simulink model "S1_DHRLs"  (R2025b)
settings: Solver=ode1be  StartTime=0.0  StopTime=0.5  RelTol=1e-3
values from neighbouring files (symbols this model uses):
  a = 10    [S1_DHRL.m]
  b = 60    [S1_DHRL.m]
  b1 = 1.2611    [S1_DHRL.m]    (also in S1_sat.m)
  b2 = 0.8909    [S1_DHRL.m]    (also in S1_sat.m)
  c1 = 15.0914    [S1_DHRL.m]    (also in S1_sat.m)
  c2 = 13.4548    [S1_DHRL.m]    (also in S1_sat.m)
  gamma = 0.5508    [S1_DHRL.m]    (also in S1_sat.m)
  h = 0.001    [S1_DHRL.m]    (also in S1_sat.m)
  k = 21.9999    [S1_DHRL.m]    (also in S1_sat.m)
  k3 = 22.5    [S1_DHRL.m]
  k4 = 7.5    [S1_DHRL.m]
  Mb = 1.999*10^-4    (= 0.0001999)    [S1_DHRL.m]    (also in S1_sat.m)
  q1 = 3    [S1_DHRL.m]
  q2 = 3    [S1_DHRL.m]
  q3 = 3    [S1_DHRL.m]
undefined symbols (not defined in the file or in its folder): magnitude
libraries: fod x6
settings Model: Creator=IT7  LastModifiedBy=Wassim DJ

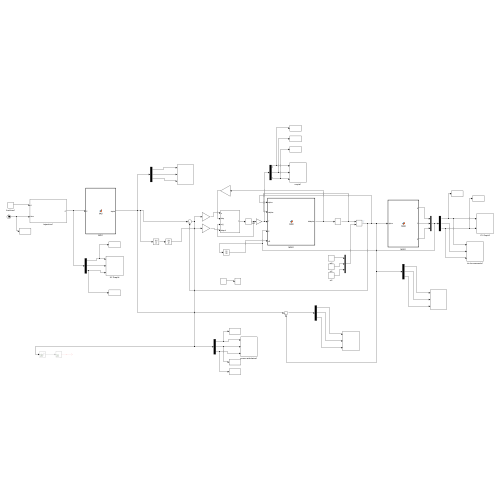
[thumbnail: Simulink's stored preview of the top-level diagram]
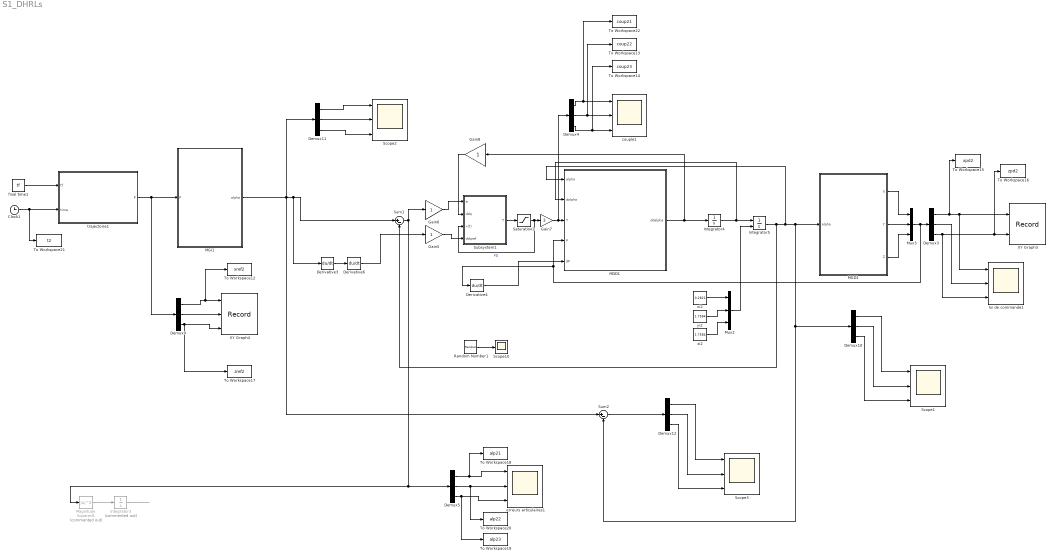
== system S1_DHRLs ==
  Clock1 : Clock
  Demux{3..5,9..12} (7 alike) : Demux  Outputs=3
  Derivative3 : Derivative
  Derivative4 : Derivative
  Derivative6 : Derivative
  Gain5 : Gain
  Gain6 : Gain
  Gain7 : Gain  Gain=3
  Gain8 : Gain
  Integrator3 : Integrator  Commented=on  InitialCondition=[0 0 0]
  Integrator4 : Integrator
  Integrator5 : Integrator  InitialConditionSource=external
  MDD1 : MATLAB Function  TreatAsAtomicUnit=on
  MGD1 : MATLAB Function  TreatAsAtomicUnit=on
  MGI1 : MATLAB Function  TreatAsAtomicUnit=on
  Magnitude Squared1 : Math  Commented=on  Operator=magnitude^2
  Mux2 : Mux  Inputs=3
  Mux3 : Mux  Inputs=3
  Random Number1 : RandomNumber  Variance=0.001  Seed=4  SampleTime=0.001
  Saturation2 : Saturate  UpperLimit=15/12  LowerLimit=-15/12
  Scope1 : Scope  NumInputPorts=3
      settings: ActiveDisplayYMinimum=-0.04767  ActiveDisplayYMaximum=2.22139
  Scope10 : Scope
      settings: ActiveDisplayYMinimum=-0.11225  ActiveDisplayYMaximum=0.1102  DataLoggingVariableName=ScopeData2
  Scope2 : Scope  NumInputPorts=3
      settings: ActiveDisplayYMinimum=-0.0501  ActiveDisplayYMaximum=2.21858  DataLoggingVariableName=ScopeData3
  Scope3 : Scope  NumInputPorts=3
      settings: ActiveDisplayYMinimum=-0.00704  ActiveDisplayYMaximum=0.00073  DataLoggingVariableName=ScopeData4
  Subsystem1 : Subsystem
  Sum1 : Sum  Inputs=|+-
  Sum2 : Sum  Inputs=|+-
  To Workspace12 : ToWorkspace  VariableName=xref2  SampleTime=-1
      settings: Save2DSignal=2-D array (concatenate along first dimension)
  To Workspace13 : ToWorkspace  VariableName=coup22  SampleTime=-1
      settings: Save2DSignal=2-D array (concatenate along first dimension)
  To Workspace14 : ToWorkspace  VariableName=coup23  SampleTime=-1
      settings: Save2DSignal=2-D array (concatenate along first dimension)
  To Workspace15 : ToWorkspace  VariableName=xpd2  SampleTime=-1
      settings: Save2DSignal=2-D array (concatenate along first dimension)
  To Workspace16 : ToWorkspace  VariableName=zpd2  SampleTime=-1
      settings: Save2DSignal=2-D array (concatenate along first dimension)
  To Workspace17 : ToWorkspace  VariableName=zref2  SampleTime=-1
      settings: Save2DSignal=2-D array (concatenate along first dimension)
  To Workspace18 : ToWorkspace  VariableName=alp21  SampleTime=-1
      settings: Save2DSignal=2-D array (concatenate along first dimension)
  To Workspace19 : ToWorkspace  VariableName=alp23  SampleTime=-1
      settings: Save2DSignal=2-D array (concatenate along first dimension)
  To Workspace20 : ToWorkspace  VariableName=alp22  SampleTime=-1
      settings: Save2DSignal=2-D array (concatenate along first dimension)
  To Workspace21 : ToWorkspace  VariableName=t2  SampleTime=-1
      settings: Save2DSignal=2-D array (concatenate along first dimension)
  To Workspace22 : ToWorkspace  VariableName=coup21  SampleTime=-1
      settings: Save2DSignal=2-D array (concatenate along first dimension)
  XY Graph3 : Record  NumPorts=2.0  FileSettingsInternal="{\"entries\":[{\"content\":{\"excelSettings\":{\"content\":{},\"type\":\"Streamout.ExcelSettings\"},\"parquetSettings\":{\"content\":{},\"type\":\"Streamout.ParquetSettings\"}},\"type\":\"Streamout.FileSettingStorage\",\"uuid\":\"\"}],\"packageUris\":[\"http:\\/\\/schema.mathworks.com\\/mf0\\/streamout_blocks\\/R2020a\"],\"version\":\"1.0\"}"  FrameSettings=[0, 0]  Layout=[1 1]  SignalsInternal="{\"entries\":[{\"content\":{\"signals\":[{\"content\":{\"blockPath\":[],\"dimensions\":[1],\"domain\":\"\",\"lineColor\":\"#edb120\",\"lineWidth\":2,\"port\":1,\"signalID\":1,\"signalName\":\"Demux3:1\"},\"type\":\"RecordBlkView.Signal\",\"uuid\":\"\"},{\"content\":{\"blockPath\":[],\"dimensions\":[1],\"domain\":\"\",\"lineColor\":\"#7e2f8e\",\"lineWidth\":2,\"port\":2,\"signalID\":2,\"signalName\":\"Demux3:3\"},\"type\":\"RecordBlkView.Signal\",\"uuid\":\"\"}]},\"type\":\"RecordBlkView.InputSignals\",\"uuid\":\"\"}],\"packageUris\":[\"http:\\/\\/schema.mathworks.com\\/mf0\\/streamout_blocks\\/R2020a\"],\"version\":\"1.0\"}"  VisualizationBindings="{\"xyplotplugin\":{\"info\":[{\"series\":[],\"subplotID\":1}]}}"  CompatibilityTag=XY  st=-1
  XY Graph4 : Record  NumPorts=3.0  FileSettingsInternal="{\"entries\":[{\"content\":{\"excelSettings\":{\"content\":{},\"type\":\"Streamout.ExcelSettings\"},\"parquetSettings\":{\"content\":{},\"type\":\"Streamout.ParquetSettings\"}},\"type\":\"Streamout.FileSettingStorage\",\"uuid\":\"\"}],\"packageUris\":[\"http:\\/\\/schema.mathworks.com\\/mf0\\/streamout_blocks\\/R2020a\"],\"version\":\"1.0\"}"  FrameSettings=[0, 0, 0]  Layout=[1 1]  SignalsInternal="{\"entries\":[{\"content\":{\"signals\":[{\"content\":{\"blockPath\":[],\"dimensions\":[1,1],\"domain\":\"\",\"lineColor\":\"#77ac30\",\"lineWidth\":2,\"port\":1,\"signalID\":1,\"signalName\":\"Demux9:1\"},\"type\":\"RecordBlkView.Signal\",\"uuid\":\"\"},{\"content\":{\"blockPath\":[],\"dimensions\":[1,1],\"domain\":\"\",\"lineColor\":\"#4dbeee\",\"lineWidth\":2,\"port\":2,\"signalID\":2,\"signalName\":\"Demux9:2\"},\"type\":\"RecordBlkView.Signal\",\"uuid\":\"\"},{\"content\":{\"blockPath\":[],\"dimensions\":[1,1],\"domain\":\"\",\"lineColor\":\"#a2142f\",\"lineWidth\":2,\"port\":3,\"signalID\":3,\"signalName\":\"Demux9:3\"},\"type\":\"RecordBlkView.Signal\",\"uuid\":\"\"}]},\"type\":\"RecordBlkView.InputSignals\",\"uuid\":\"\"}],\"packageUris\":[\"http:\\/\\/schema.mathworks.com\\/mf0\\/streamout_blocks\\/R2020a\"],\"version\":\"1.0\"}"  VisualizationBindings="{\"xyplotplugin\":{\"info\":[{\"series\":[],\"subplotID\":1}]}}"  CompatibilityTag=XY  st=-1
  couple1 : Scope  NumInputPorts=3
      settings: ActiveDisplayYMinimum=-10.50451  ActiveDisplayYMaximum=10.07629  DataLoggingVariableName=ScopeData5
  erreurs articulaires1 : Scope  NumInputPorts=3
      settings: ActiveDisplayYMinimum=-0.00893  ActiveDisplayYMaximum=0.00194  DataLoggingVariableName=ScopeData6
  final time1 : Constant  Value=tf
  loi de commande1 : Scope  NumInputPorts=3
      settings: ActiveDisplayYMinimum=-0.50497  ActiveDisplayYMaximum=0.51496
  trajectoire1 : Subsystem
  xi2 : Constant  Value=0.2821
  yi2 : Constant  Value=1.7584
  zi2 : Constant  Value=1.7584
  wires:
  Integrator3/1 -> ?
  Demux12/2 -> Scope3/2
  xi2/1 -> Mux2/1
  Demux11/3 -> Scope2/3
  yi2/1 -> Mux2/2
  Subsystem1/1(T) -> Saturation2/1
  Demux12/3 -> Scope3/3
  Demux10/3 -> Scope1/3
  Demux3/1 -> XY Graph3/1, loi de commande1/1, To Workspace15/1
  Demux5/2 -> To Workspace20/1, erreurs articulaires1/2
  Demux4/1 -> To Workspace22/1, couple1/1
  Gain5/1 -> Subsystem1/4(ddqref)
  Gain8/1 -> Subsystem1/2(ddq)
  Derivative6/1 -> Gain5/1
  Mux2/1 -> Integrator5/2
  Derivative4/1 -> MDD1/5(dP)
  Random Number1/1 -> Scope10/1
  zi2/1 -> Mux2/3
  Sum2/1 -> Demux12/1
  Demux11/2 -> Scope2/2
  Gain7/1 -> Demux4/1, MDD1/3(T)
  Demux9/3 -> XY Graph4/3, To Workspace17/1
  trajectoire1/1(P) -> Demux9/1, MGI1/1(P)
  Demux9/1 -> To Workspace12/1, XY Graph4/1
  Demux11/1 -> Scope2/1
  Demux5/1 -> To Workspace18/1, erreurs articulaires1/1
  Derivative3/1 -> Derivative6/1
  final time1/1 -> trajectoire1/1(tf)
  Demux10/2 -> Scope1/2
  Integrator5/1 -> Sum1/2, MDD1/1(alpha), MGD1/1(alpha), Demux10/1, Sum2/2
  MDD1/1(ddalpha) -> Gain8/1, Integrator4/1
  MGD1/2(Y) -> Mux3/2
  MGD1/1(X) -> Mux3/1
  MGI1/1(alpha) -> Derivative3/1, Sum1/1, Sum2/1, Demux11/1
  Saturation2/1 -> Subsystem1/3(x(t)), Gain7/1  "PD"
  Demux9/2 -> XY Graph4/2
  Integrator4/1 -> MDD1/2(dalpha), Integrator5/1
  Demux4/3 -> To Workspace14/1, couple1/3
  Demux4/2 -> To Workspace13/1, couple1/2
  Demux10/1 -> Scope1/1
  Sum1/1 -> Magnitude Squared1/1, Demux5/1, Gain6/1
  Demux3/2 -> loi de commande1/2
  Magnitude Squared1/1 -> Integrator3/1
  Clock1/1 -> To Workspace21/1, trajectoire1/2("time ")
  Gain6/1 -> Subsystem1/1(e)
  MGD1/3(Z) -> Mux3/3
  Demux3/3 -> loi de commande1/3, XY Graph3/2, To Workspace16/1
  Mux3/1 -> MDD1/4(P), Derivative4/1, Demux3/1
  Demux5/3 -> To Workspace19/1, erreurs articulaires1/3
  Demux12/1 -> Scope3/1

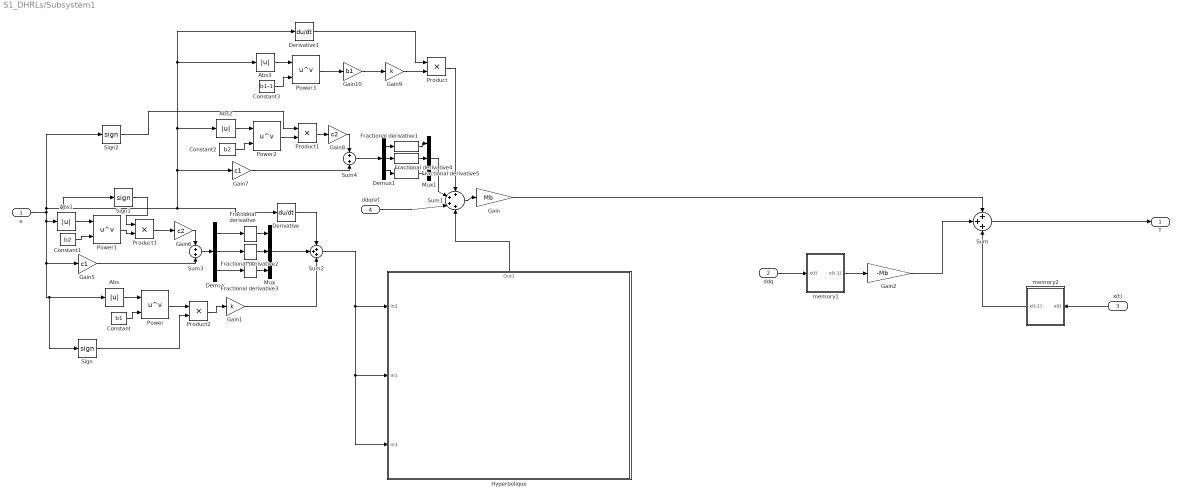
== system S1_DHRLs/Subsystem1 ==
  e : Inport
  ddq : Inport  Port=2
  x(t) : Inport  Port=3
  ddqref : Inport  Port=4
  Abs{,1..3} (4 alike) : Abs  SaturateOnIntegerOverflow=off
  Constant : Constant  Value=b1
  Constant1 : Constant  Value=b2
  Constant2 : Constant  Value=b2
  Constant3 : Constant  Value=b1-1
  Demux : Demux  Outputs=3
  Demux1 : Demux  Outputs=3
  Derivative : Derivative
  Derivative1 : Derivative
  Fractional derivative : fod/Fractional derivative  gam=gamma  ww=[0.001; 1000]  n=5  nFod=off
      settings: SourceProductName=FOMCON Toolbox
  Fractional derivative1 : fod/Fractional derivative  gam=gamma+1  ww=[0.001; 1000]  n=5  nFod=off
      settings: SourceProductName=FOMCON Toolbox
  Fractional derivative2 : fod/Fractional derivative  gam=gamma  ww=[0.001; 1000]  n=5  nFod=off
      settings: SourceProductName=FOMCON Toolbox
  Fractional derivative3 : fod/Fractional derivative  gam=gamma  ww=[0.001; 1000]  n=5  nFod=off
      settings: SourceProductName=FOMCON Toolbox
  Fractional derivative4 : fod/Fractional derivative  gam=gamma+1  ww=[0.001; 1000]  n=5  nFod=off
      settings: SourceProductName=FOMCON Toolbox
  Fractional derivative5 : fod/Fractional derivative  gam=gamma+1  ww=[0.001; 1000]  n=5  nFod=off
      settings: SourceProductName=FOMCON Toolbox
  Gain : Gain  Gain=Mb
  Gain1 : Gain  Gain=k
  Gain10 : Gain  Gain=b1
  Gain2 : Gain  Gain=-Mb
  Gain5 : Gain  Gain=c1
  Gain6 : Gain  Gain=c2
  Gain7 : Gain  Gain=c1
  Gain8 : Gain  Gain=c2
  Gain9 : Gain  Gain=k
  Hyperbolique : Subsystem
      settings: PortSchema="{\"entries\":[{\"content\":{\"sides\":[{\"content\":{\"connectorIds\":[\"In1\",\"In2\",\"In3\"]},\"type\":\"ConnectorPlacement.EquallySpacedRectSide\",\"uuid\":\"207838c6-2501-4f04-97a9-df665208479a\"},{\"content\":{\"side\":\"RIGHT\"},\"type\":\"ConnectorPlacement.EquallySpacedRectSide\",\"uuid\":\"24f737b7-daa2-4ae5-8b85-6b96e3603981\"},{\"content\":{\"connectorIds\":[\"Out1\"],\"side\":\"TOP\"},\"type\":\"ConnectorPlacement.EquallySpacedRectSide\",\"uuid\":\"32365517-b7f0-439b-b759-bae0c7d72860\"}]},\"type\":\"ConnectorPlacement.EquallySpacedConnector\",\"uuid\":\"217bfbcb-c426-4fed-87a9-fb4c75bdc6df\"}],\"packageUris\":[\"http://schema.mathworks.com/mf0/Connector/R2020b\"],\"version\":\"1.0\"}"
  Mux : Mux  Inputs=3
  Mux1 : Mux  Inputs=3
  Power{,1..3} (4 alike) : Math  Operator=pow
  Product{,1..3} (4 alike) : Product
  Sign : Signum
  Sign1 : Signum
  Sign2 : Signum
  Sum : Sum  Inputs=+++
  Sum1 : Sum  Inputs=++++
  Sum2 : Sum  Inputs=+++
  Sum3 : Sum
  Sum4 : Sum
  memory1 : Subsystem
  memory2 : Subsystem
  T : Outport  VectorParamsAs1DForOutWhenUnconnected=off
  wires:
  Derivative/1 -> Sum2/1
  Sum1/1 -> Gain/1
  Sum/1 -> T/1
  Gain/1 -> Sum/1
  Abs/1 -> Power/1
  Constant/1 -> Power/2
  Power/1 -> Product2/1
  Gain1/1 -> Sum2/3
  Constant1/1 -> Power1/2
  Abs1/1 -> Power1/1
  Gain5/1 -> Sum3/2
  Gain6/1 -> Sum3/1
  Abs2/1 -> Power2/1
  Gain8/1 -> Sum4/1
  Power2/1 -> Product1/2
  Product1/1 -> Gain8/1
  Gain7/1 -> Sum4/2
  Constant2/1 -> Power2/2
  Abs3/1 -> Power3/1
  Power3/1 -> Gain10/1
  Gain10/1 -> Gain9/1
  Constant3/1 -> Power3/2
  Product/1 -> Sum1/1
  Gain9/1 -> Product/2
  Derivative1/1 -> Product/1
  Sum3/1 -> Demux/1
  Demux/1 -> Fractional derivative/1
  Demux/2 -> Fractional derivative2/1
  Demux/3 -> Fractional derivative3/1
  Fractional derivative/1 -> Mux/1
  Fractional derivative3/1 -> Mux/3
  Fractional derivative2/1 -> Mux/2
  Mux/1 -> Sum2/2
  Sum4/1 -> Demux1/1
  Demux1/1 -> Fractional derivative1/1
  Fractional derivative1/1 -> Mux1/1
  Fractional derivative4/1 -> Mux1/2
  Demux1/2 -> Fractional derivative4/1
  Fractional derivative5/1 -> Mux1/3
  Demux1/3 -> Fractional derivative5/1
  Sign2/1 -> Product1/1
  Product2/1 -> Gain1/1
  Sign/1 -> Product2/2
  Product3/1 -> Gain6/1
  Power1/1 -> Product3/2
  Sign1/1 -> Product3/1
  Mux1/1 -> Sum1/2
  e/1 -> Abs1/1, Sign/1, Abs/1, Gain5/1, Sign2/1, Sign1/1, Abs3/1, Derivative1/1, Abs2/1, Gain7/1, Derivative/1
  ddqref/1 -> Sum1/3
  Hyperbolique/1(Out1) -> Sum1/4
  Sum2/1 -> Hyperbolique/1(In2), Hyperbolique/3(In3), Hyperbolique/2(In1)
  ddq/1 -> memory1/1(x(t))
  x(t)/1 -> memory2/1(x(t))
  Gain2/1 -> Sum/2
  memory1/1(x(t-1)) -> Gain2/1
  memory2/1(x(t-1)) -> Sum/3

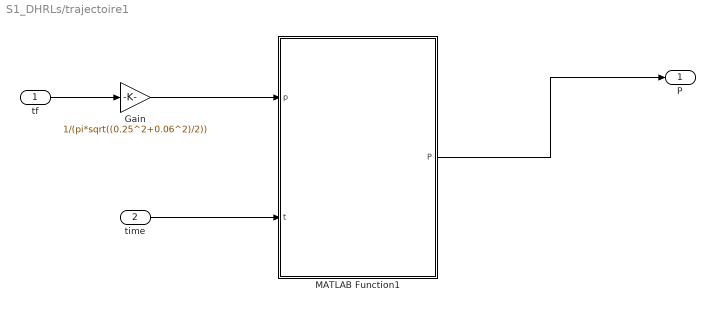
== system S1_DHRLs/trajectoire1 ==
  tf : Inport
  "time " : Inport  Port=2
  Gain : Gain  Gain=1/(pi*sqrt((0.25^2+0.06^2)/2))
  MATLAB Function1 : MATLAB Function  TreatAsAtomicUnit=on
  P : Outport  VectorParamsAs1DForOutWhenUnconnected=off
  wires:
  MATLAB Function1/1(P) -> P/1
  Gain/1 -> MATLAB Function1/1(p)
  "time "/1 -> MATLAB Function1/2(t)
  tf/1 -> Gain/1

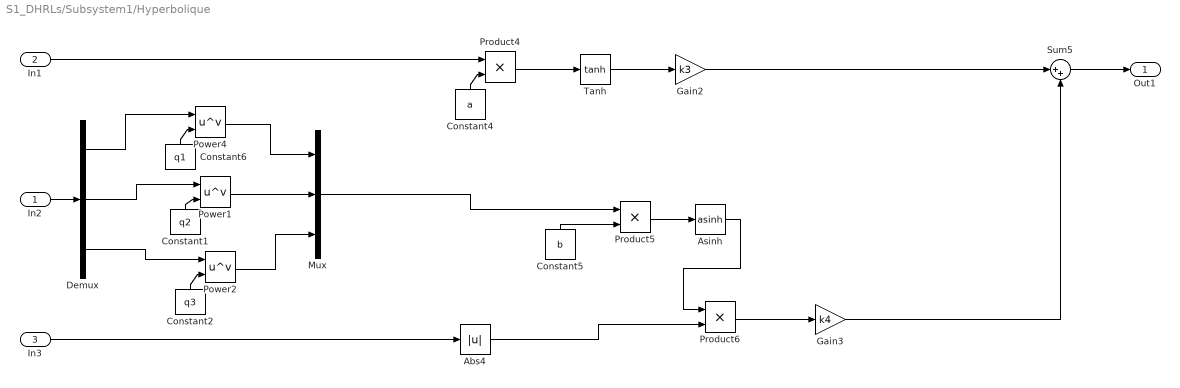
== system S1_DHRLs/Subsystem1/Hyperbolique ==
  In2 : Inport
  In1 : Inport  Port=2
  In3 : Inport  Port=3
  Abs4 : Abs  SaturateOnIntegerOverflow=off
  Asinh : Trigonometry  Operator=asinh
  Constant1 : Constant  Value=q2
  Constant2 : Constant  Value=q3
  Constant4 : Constant  Value=a
  Constant5 : Constant  Value=b
  Constant6 : Constant  Value=q1
  Demux : Demux  Outputs=3
  Gain2 : Gain  Gain=k3
  Gain3 : Gain  Gain=k4
  Mux : Mux  Inputs=3
  Power1 : Math  Operator=pow
  Power2 : Math  Operator=pow
  Power4 : Math  Operator=pow
  Product4 : Product
  Product5 : Product
  Product6 : Product
  Sum5 : Sum  Inputs=|++
  Tanh : Trigonometry  Operator=tanh
  Out1 : Outport
  wires:
  Abs4/1 -> Product6/2
  Product4/1 -> Tanh/1
  Constant5/1 -> Product5/2
  Constant6/1 -> Power4/2
  Constant4/1 -> Product4/2
  Product5/1 -> Asinh/1
  Asinh/1 -> Product6/1
  Sum5/1 -> Out1/1
  In3/1 -> Abs4/1
  In1/1 -> Product4/1
  Constant1/1 -> Power1/2
  Constant2/1 -> Power2/2
  In2/1 -> Demux/1
  Demux/1 -> Power4/1
  Demux/2 -> Power1/1
  Demux/3 -> Power2/1
  Power1/1 -> Mux/2
  Power4/1 -> Mux/1
  Power2/1 -> Mux/3
  Mux/1 -> Product5/1
  Product6/1 -> Gain3/1
  Gain3/1 -> Sum5/2
  Tanh/1 -> Gain2/1
  Gain2/1 -> Sum5/1

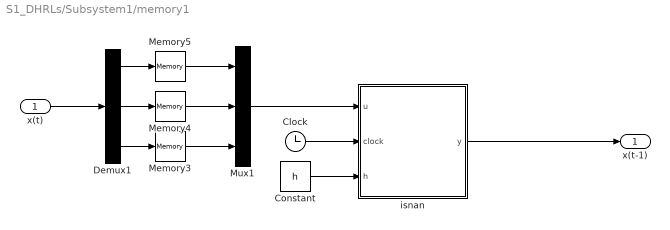
== system S1_DHRLs/Subsystem1/memory1 ==
  x(t) : Inport
  Clock : Clock
  Constant : Constant  Value=h
  Demux1 : Demux  Outputs=3
  Memory3 : Memory
  Memory4 : Memory
  Memory5 : Memory
  Mux1 : Mux  Inputs=3
  isnan : MATLAB Function  TreatAsAtomicUnit=on
  x(t-1) : Outport  VectorParamsAs1DForOutWhenUnconnected=off
  wires:
  x(t)/1 -> Demux1/1
  Demux1/1 -> Memory5/1
  Demux1/3 -> Memory3/1
  Demux1/2 -> Memory4/1
  Memory5/1 -> Mux1/1
  Memory4/1 -> Mux1/2
  Memory3/1 -> Mux1/3
  Mux1/1 -> isnan/1(u)
  isnan/1(y) -> x(t-1)/1
  Clock/1 -> isnan/2(clock)
  Constant/1 -> isnan/3(h)

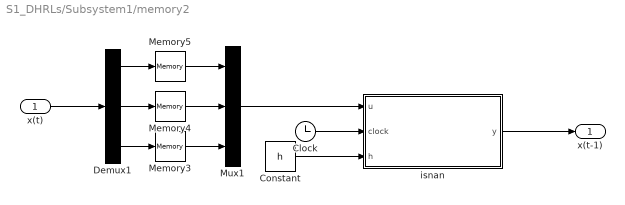
== system S1_DHRLs/Subsystem1/memory2 ==
  x(t) : Inport
  Clock : Clock
  Constant : Constant  Value=h
  Demux1 : Demux  Outputs=3
  Memory3 : Memory  InheritSampleTime=on
  Memory4 : Memory  InheritSampleTime=on
  Memory5 : Memory  InheritSampleTime=on
  Mux1 : Mux  Inputs=3
  isnan : MATLAB Function  TreatAsAtomicUnit=on
  x(t-1) : Outport  VectorParamsAs1DForOutWhenUnconnected=off
  wires:
  x(t)/1 -> Demux1/1
  Demux1/1 -> Memory5/1
  Demux1/3 -> Memory3/1
  Demux1/2 -> Memory4/1
  Memory5/1 -> Mux1/1
  Memory4/1 -> Mux1/2
  Memory3/1 -> Mux1/3
  Mux1/1 -> isnan/1(u)
  isnan/1(y) -> x(t-1)/1
  Clock/1 -> isnan/2(clock)
  Constant/1 -> isnan/3(h)

== matlab function S1_DHRLs/MDD1 ==
  data: alpha input; ddalpha output; dalpha input; T input; P input; dP input
function ddalpha = MDD(alpha,dalpha,T,P,dP)
ddalpha = zeros(1,3);
phi = [0 2*pi/3 4*pi/3];
l1 = 0.205;
r = 0.15-0.024;
% these boudjedir table 2.1 page 30
mn = 0.042;
mfb = 0.028;
mb = 0.098;
mc = 0.015;
g = 9.81;
Im = 3.72e-5;
% mch=0.7;
% documentation 0
% rotation matrix
R1 = [cos(phi(1)) -sin(phi(1)) 0;sin(phi(1)) cos(phi(1)) 0;0 0 1];
R2 = [cos(phi(2)) -sin(phi(2)) 0;sin(phi(2)) cos(phi(2)) 0;0 0 1]; 
R3 = [cos(phi(3)) -sin(phi(3)) 0;sin(phi(3)) cos(phi(3)) 0;0 0 1]; 

% eq 4.4
s1 = [P(1);P(2);P(3)]-R1*([r;0;0]+[l1*cos(alpha(1));0;l1*sin(alpha(1))]);    
s2 = [P(1);P(2);P(3)]-R2*([r;0;0]+[l1*cos(alpha(2));0;l1*sin(alpha(2))]); 
s3 = [P(1);P(2);P(3)]-R3*([r;0;0]+[l1*cos(alpha(3));0;l1*sin(alpha(3))]); 

% eq 4.9
b1 = R1*[-l1*sin(alpha(1));0;l1*cos(alpha(1))];
b2 = R2*[-l1*sin(alpha(2));0;l1*cos(alpha(2))];
b3 = R3*[-l1*sin(alpha(3));0;l1*cos(alpha(3))];

% eq 4.8
ds1 = [dP(1);dP(2);dP(3)]-R1*[-l1*sin(alpha(1));0;l1*cos(alpha(1))]*dalpha(1);
ds2 = [dP(1);dP(2);dP(3)]-R2*[-l1*sin(alpha(2));0;l1*cos(alpha(2))]*dalpha(2);
ds3 = [dP(1);dP(2);dP(3)]-R3*[-l1*sin(alpha(3));0;l1*cos(alpha(3))]*dalpha(3);

db1 = R1*[-l1*cos(alpha(1));0;-l1*sin(alpha(1))]*dalpha(1);
db2 = R2*[-l1*cos(alpha(2));0;-l1*sin(alpha(2))]*dalpha(2);
db3 = R3*[-l1*cos(alpha(3));0;-l1*sin(alpha(3))]*dalpha(3);

% eq 4.13
J = inv([s1';s2';s3'])*[s1'*b1 0 0;0 s2'*b2 0;0 0 s3'*b3];

dJ = inv([s1';s2';s3'])*(-[ds1';ds2';ds3']*J+[ds1'*b1+s1'*db1 0 0;0 ds2'*b2+s2'*db2 0;0 0 ds3'*b3+s3'*db3]);
% these boudjedir
% equa 2.42
mnt = mn+mfb; %+mch

% equa 2.49
Tgn = J'*mnt*[0 0 -g]';

% equa 2.44
mbr = mb+mc+2/3*mfb;

% equa 2.43
rgb = l1*(1/2*mb+mc+2/3*mfb)/mbr;

% equa 2.50
Tgb = rgb*mbr*g*[cos(alpha(1)) cos(alpha(2)) cos(alpha(3))]';

% equa 2.46
Ibc = l1^2*(mb/3+mc+2/3*mfb);
% equa 2.45
Ib = (Im*12^2+Ibc)*eye(3);

% equa 2.54
 ddalpha = (inv(Ib + mnt*J'*J)*(T - J'*mnt*dJ*dalpha' + Tgn + Tgb))';
if isnan(ddalpha)
    ddalpha = zeros(1,3);
end

== matlab function S1_DHRLs/MGD1 ==
  data: alpha input; X output; Y output; Z output
function [X,Y,Z]  = MGD(alpha)

phi = [0 2*pi/3 4*pi/3];
l1 = 0.205;
l2 = 0.380;
r = 0.15-0.024;

D = zeros(1,3);
E = zeros(1,3);
F = zeros(1,3);
G = zeros(1,3);

for i=1:3
   D(i)=-l2^2+l1^2+r^2+2*r*l1*cos(alpha(i));
   E(i)=2*(r+l1*cos(alpha(i)))*cos(phi(i));
   F(i)=2*(r+l1*cos(alpha(i)))*sin(phi(i));
   G(i)=-2*l1*sin(alpha(i))  ;
end
% H1 = -(E(3)-E(1))*(G(2)-G(1))+(G(3)-G(1))*(E(2)-E(1));
% H2 = -(F(3)-F(1))*(E(2)-E(1))+(E(3)-E(1))*(F(2)-F(1));
% H3 = -(D(3)-D(1))*(E(2)-E(1))+(E(3)-E(1))*(D(2)-D(1));
% H4 = (D(3)-D(1))*(F(2)-F(1))-(F(3)-F(1))*(D(1)-D(2));
% H5 = -(G(3)-G(1))*(F(2)-F(1))-(F(3)-F(1))*(G(1)-G(2));

H1 = E(1)*G(2)-E(1)*G(3)-E(2)*G(1)+E(2)*G(3)+E(3)*G(1)-E(3)*G(2);
H2 = E(1)*(-F(2)+F(3))+E(2)*(F(1)-F(3))+E(3)*(-F(1)+F(2));
H3 = E(1)*(-D(2)+D(3))+E(2)*(D(1)-D(3))+E(3)*(-D(1)+D(2));
H4 = F(1)*(D(2)-D(3))+F(2)*(-D(1)+D(3))+F(3)*(D(1)-D(2));
H5 = F(1)*(-G(2)+G(3))+F(2)*(G(1)-G(3))+F(3)*(-G(1)+G(2));

L = ((H5^2+H1^2)/(H2^2))+1;
M = 2*(H5*H4+H1*H3)/(H2^2)-(H5*E(1)+H1*F(1))/H2-G(1);
N = (H4^2+H3^2)/H2^2-(H4*E(1)+H3*F(1))/H2+D(1);
Z = min((-M+sqrt(abs(M^2-4*L*N)))/(2*L),(-M-sqrt(abs(M^2-4*L*N)))/(2*L));
X = Z*(H5/H2)+(H4/H2);
Y = Z*(H1/H2)+(H3/H2);

X = double(X);
Y = double(Y);
Z = double(Z);

== matlab function S1_DHRLs/MGI1 ==
  data: P input; alpha output
function alpha = MGI(P)
phi = [0 2*pi/3 4*pi/3];
l1 = 0.205;
l2 = 0.380;
r = 0.15-0.024;
X = P(1,1);
Y = P(1,2);
Z = P(1,3);

A = zeros(1,3);
B = 2*Z*l1;
C = zeros(1,3);

for i=1:3
A(i) = 2*r*l1-2*X*l1*cos(phi(i))-2*Y*l1*sin(phi(i));
C(i) = l2^2-l1^2-r^2-X^2-Y^2-Z^2+2*X*r*cos(phi(i))+2*Y*r*sin(phi(i));    
end

alpha = zeros(1,3);
for i=1:3
    alpha(i) =  2*atan( (2*B+sqrt(abs(4*B^2+4*(A(i)+C(i))*(A(i)-C(i)))))/(2*(A(i)+C(i))));
    alpha(i) = double(alpha(i));
end

== matlab function S1_DHRLs/Subsystem1/memory1/isnan ==
  data: u input; y output; clock input; h input
function y = fcn(u,clock,h)
y = zeros(length(u),1);
for i = 1:3
if isnan(u(i)) || clock/h < 3
    y(i) = 0; 
else 
   y(i) = u(i);
end
end

== matlab function S1_DHRLs/Subsystem1/memory2/isnan ==
  data: u input; y output; clock input; h input
function y = fcn(u,clock,h)
y = zeros(length(u),1);
for i = 1:3
if isnan(u(i)) || clock/h < 3
    y(i) = 0; 
else 
   y(i) = u(i);
end
end

== matlab function S1_DHRLs/trajectoire1/MATLAB Function1 ==
  data: P output; p input; t input
function P   = trajectoire(p,t)


A=0.25;
B=0.06;
D=pi*sqrt((A^2+B^2)/2);



Xdes=0.25-A*(1-cos(pi*(t)/(p*D)));
Ydes=0*t;
Zdes=-0.43+B*sin(pi*(t)/(p*D));

dXdes=-A*pi/(p*D)*(sin(pi*(t)/(p*D)));
dYdes=0*t;
dZdes=B*pi/(p*D)*cos(pi*(t)/(p*D));

ddXdes=A*pi/(p*D)*pi/(p*D)*cos(pi*(t)/(p*D));
ddYdes=0*t;
ddZdes=-B*pi/(p*D)*pi/(p*D)*sin(pi*(t)/(p*D));

% Xdes=-0.25+A*(1-cos(pi*t/(p*D)));
% Ydes=0*t;
% Zdes=-0.43+B*sin(pi*t/(p*D));

P = [Xdes,Ydes,Zdes];
%dP = [dXdes,dYdes,dZdes];
%ddP = [ddXdes,ddYdes,ddZdes];

end
